simulink model "ThdRwRtStCalib"  (R2024b)
settings: Solver=FixedStepDiscrete  StartTime=0.0  StopTime=10.0  FixedStep=0.01  RelTol=1e-3
model workspace (MAT data in the model file):
  KeSMSwAcsMd7ThdRwRtStBkReclnUpwdDnwdPosMax_Val : Simulink.Parameter (value not decoded)
  KeSMSwAcsMd7ThdRwRtStBkReclnUpwdDnwdPosMin_Val : Simulink.Parameter (value not decoded)
  KeSMSwAcsMd7ThdRwRtStBkReclnUpwdDnwdPos_Val : Simulink.Parameter (value not decoded)
  KeSMSwAcsMd7ThdRwRtStCshnFldUpwdDnwdPosMax_Val : Simulink.Parameter (value not decoded)
  KeSMSwAcsMd7ThdRwRtStCshnFldUpwdDnwdPosMin_Val : Simulink.Parameter (value not decoded)
  KeSMSwAcsMd7ThdRwRtStCshnFldUpwdDnwdPos_Val : Simulink.Parameter (value not decoded)
  KeSMSwAcsMd7ThdRwRtStFrwdBkwdPosMax_Val : Simulink.Parameter (value not decoded)
  KeSMSwAcsMd7ThdRwRtStFrwdBkwdPosMin_Val : Simulink.Parameter (value not decoded)
  KeSMSwAcsMd7ThdRwRtStFrwdBkwdPos_Val : Simulink.Parameter (value not decoded)
symbols that are objects in the model workspace (value not decoded): KeSMSwAcsMd7ThdRwRtStBkReclnUpwdDnwdPos_Val, KeSMSwAcsMd7ThdRwRtStBkReclnUpwdDnwdPosMax_Val, KeSMSwAcsMd7ThdRwRtStBkReclnUpwdDnwdPosMin_Val, KeSMSwAcsMd7ThdRwRtStCshnFldUpwdDnwdPos_Val, KeSMSwAcsMd7ThdRwRtStCshnFldUpwdDnwdPosMax_Val, KeSMSwAcsMd7ThdRwRtStCshnFldUpwdDnwdPosMin_Val, KeSMSwAcsMd7ThdRwRtStFrwdBkwdPos_Val, KeSMSwAcsMd7ThdRwRtStFrwdBkwdPosMax_Val, KeSMSwAcsMd7ThdRwRtStFrwdBkwdPosMin_Val
undefined symbols (not defined in the file or in its folder): KeSMSw6sAcsEntryThdRwRtStBkReclnUpwdDnwdPos_Val, KeSMSw6sAcsEntryThdRwRtStBkReclnUpwdDnwdPosMax_Val, KeSMSw6sAcsEntryThdRwRtStBkReclnUpwdDnwdPosMin_Val, KeSMSw6sAcsEntryThdRwRtStCshnFldUpwdDnwdPos_Val, KeSMSw6sAcsEntryThdRwRtStCshnFldUpwdDnwdPosMax_Val, KeSMSw6sAcsEntryThdRwRtStCshnFldUpwdDnwdPosMin_Val, KeSMSw6sAcsEntryThdRwRtStFrwdBkwdPos_Val, KeSMSw6sAcsEntryThdRwRtStFrwdBkwdPosMax_Val, KeSMSw6sAcsEntryThdRwRtStFrwdBkwdPosMin_Val, KeSMSw6SAcsMd56ThdRwRtStBkReclnUpwdDnwdPos_Val, KeSMSw6SAcsMd56ThdRwRtStBkReclnUpwdDnwdPosMax_Val, KeSMSw6SAcsMd56ThdRwRtStBkReclnUpwdDnwdPosMin_Val, KeSMSw6SAcsMd56ThdRwRtStFrwdBkwdPos_Val, KeSMSw6SAcsMd56ThdRwRtStFrwdBkwdPosMax_Val, KeSMSw6SAcsMd56ThdRwRtStFrwdBkwdPosMin_Val, KeSMSw6SAcsMd57ThdRwRtStBkReclnUpwdDnwdPos_Val, KeSMSw6SAcsMd57ThdRwRtStBkReclnUpwdDnwdPosMax_Val, KeSMSw6SAcsMd57ThdRwRtStBkReclnUpwdDnwdPosMin_Val, KeSMSw6SAcsMd57ThdRwRtStFrwdBkwdPos_Val, KeSMSw6SAcsMd57ThdRwRtStFrwdBkwdPosMax_Val, KeSMSw6SAcsMd57ThdRwRtStFrwdBkwdPosMin_Val, KeSMSw6sFamilyMdThdRwRtStFrwdBkwdPos_Val, KeSMSw6sFamilyMdThdRwRtStFrwdBkwdPosMax_Val, KeSMSw6sFamilyMdThdRwRtStFrwdBkwdPosMin_Val, KeSMSw6sFamilyRMdThdRwRtStFrwdBkwdPos_Val, KeSMSw6sFamilyRMdThdRwRtStFrwdBkwdPosMax_Val, KeSMSw6sFamilyRMdThdRwRtStFrwdBkwdPosMin_Val, KeSMSw6sLugThdRwRtStBkReclnUpwdDnwdPos_Val, KeSMSw6sLugThdRwRtStBkReclnUpwdDnwdPosMax_Val, KeSMSw6sLugThdRwRtStBkReclnUpwdDnwdPosMin_Val, KeSMSw6sLugThdRwRtStCshnFldUpwdDnwdPos_Val, KeSMSw6sLugThdRwRtStCshnFldUpwdDnwdPosMax_Val, KeSMSw6sLugThdRwRtStCshnFldUpwdDnwdPosMin_Val, KeSMSw6sLugThdRwRtStFrwdBkwdPos_Val, KeSMSw6sLugThdRwRtStFrwdBkwdPosMax_Val, KeSMSw6sLugThdRwRtStFrwdBkwdPosMin_Val, KeSMSw6sVIPThdRwRtStBkReclnUpwdDnwdPos_Val, KeSMSw6sVIPThdRwRtStBkReclnUpwdDnwdPosMax_Val, KeSMSw6sVIPThdRwRtStBkReclnUpwdDnwdPosMin_Val, KeSMSw6sVIPThdRwRtStFrwdBkwdPos_Val, KeSMSw6sVIPThdRwRtStFrwdBkwdPosMax_Val, KeSMSw6sVIPThdRwRtStFrwdBkwdPosMin_Val, KeSMSwAcsEntryThdRwRtStBkReclnUpwdDnwdPos_Val, KeSMSwAcsEntryThdRwRtStBkReclnUpwdDnwdPosMax_Val, KeSMSwAcsEntryThdRwRtStBkReclnUpwdDnwdPosMin_Val, KeSMSwAcsEntryThdRwRtStCshnFldUpwdDnwdPos_Val, KeSMSwAcsEntryThdRwRtStCshnFldUpwdDnwdPosMax_Val, KeSMSwAcsEntryThdRwRtStCshnFldUpwdDnwdPosMin_Val, KeSMSwAcsEntryThdRwRtStFrwdBkwdPos_Val, KeSMSwAcsEntryThdRwRtStFrwdBkwdPosMax_Val, KeSMSwAcsEntryThdRwRtStFrwdBkwdPosMin_Val, KeSMSwAcsMd53ThdRwRtBkReclnUpwdDnwdPos_Val, KeSMSwAcsMd53ThdRwRtBkReclnUpwdDnwdPosMax_Val, KeSMSwAcsMd53ThdRwRtBkReclnUpwdDnwdPosMin_Val, KeSMSwAcsMd53ThdRwRtFldUpwdDnwdPos_Val, KeSMSwAcsMd53ThdRwRtFldUpwdDnwdPosMax_Val, KeSMSwAcsMd53ThdRwRtFldUpwdDnwdPosMin_Val, KeSMSwAcsMd56ThdRwRtStBkReclnUpwdDnwdPos_Val, KeSMSwAcsMd56ThdRwRtStBkReclnUpwdDnwdPosMax_Val, KeSMSwAcsMd56ThdRwRtStBkReclnUpwdDnwdPosMin_Val ... (+33)
libraries: TrgtPosSelcLib x18
(part 3 of 3)

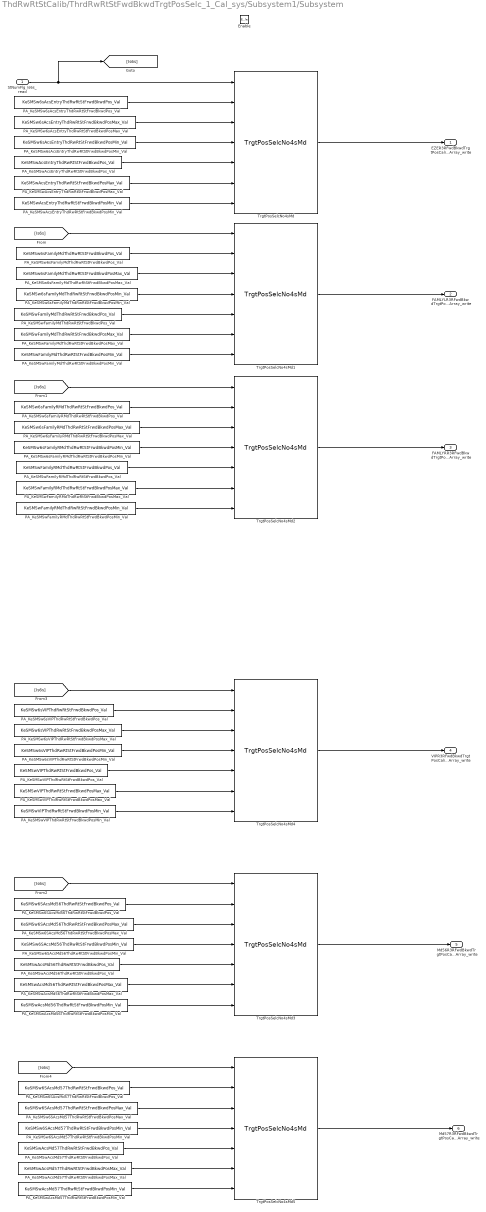
== system ThdRwRtStCalib/ThrdRwRtStFwdBkwdTrgtPosSelc_1_Cal_sys/Subsystem1/Subsystem ==
  StNumFlg_Is6s_read : Inport
  Enable : EnablePort
  PA_KeSMSw6SAcsMd56ThdRwRtStFrwdBkwdPosMax_Val : Constant  Value=KeSMSw6SAcsMd56ThdRwRtStFrwdBkwdPosMax_Val
  PA_KeSMSw6SAcsMd56ThdRwRtStFrwdBkwdPosMin_Val : Constant  Value=KeSMSw6SAcsMd56ThdRwRtStFrwdBkwdPosMin_Val
  PA_KeSMSw6SAcsMd56ThdRwRtStFrwdBkwdPos_Val : Constant  Value=KeSMSw6SAcsMd56ThdRwRtStFrwdBkwdPos_Val
  PA_KeSMSw6SAcsMd57ThdRwRtStFrwdBkwdPosMax_Val : Constant  Value=KeSMSw6SAcsMd57ThdRwRtStFrwdBkwdPosMax_Val
  PA_KeSMSw6SAcsMd57ThdRwRtStFrwdBkwdPosMin_Val : Constant  Value=KeSMSw6SAcsMd57ThdRwRtStFrwdBkwdPosMin_Val
  PA_KeSMSw6SAcsMd57ThdRwRtStFrwdBkwdPos_Val : Constant  Value=KeSMSw6SAcsMd57ThdRwRtStFrwdBkwdPos_Val
  PA_KeSMSw6sAcsEntryThdRwRtStFrwdBkwdPosMax_Val : Constant  Value=KeSMSw6sAcsEntryThdRwRtStFrwdBkwdPosMax_Val
  PA_KeSMSw6sAcsEntryThdRwRtStFrwdBkwdPosMin_Val : Constant  Value=KeSMSw6sAcsEntryThdRwRtStFrwdBkwdPosMin_Val
  PA_KeSMSw6sAcsEntryThdRwRtStFrwdBkwdPos_Val : Constant  Value=KeSMSw6sAcsEntryThdRwRtStFrwdBkwdPos_Val
  PA_KeSMSw6sFamilyMdThdRwRtStFrwdBkwdPosMax_Val : Constant  Value=KeSMSw6sFamilyMdThdRwRtStFrwdBkwdPosMax_Val
  PA_KeSMSw6sFamilyMdThdRwRtStFrwdBkwdPosMin_Val : Constant  Value=KeSMSw6sFamilyMdThdRwRtStFrwdBkwdPosMin_Val
  PA_KeSMSw6sFamilyMdThdRwRtStFrwdBkwdPos_Val : Constant  Value=KeSMSw6sFamilyMdThdRwRtStFrwdBkwdPos_Val
  PA_KeSMSw6sFamilyRMdThdRwRtStFrwdBkwdPosMax_Val : Constant  Value=KeSMSw6sFamilyRMdThdRwRtStFrwdBkwdPosMax_Val
  PA_KeSMSw6sFamilyRMdThdRwRtStFrwdBkwdPosMin_Val : Constant  Value=KeSMSw6sFamilyRMdThdRwRtStFrwdBkwdPosMin_Val
  PA_KeSMSw6sFamilyRMdThdRwRtStFrwdBkwdPos_Val : Constant  Value=KeSMSw6sFamilyRMdThdRwRtStFrwdBkwdPos_Val
  PA_KeSMSw6sVIPThdRwRtStFrwdBkwdPosMax_Val : Constant  Value=KeSMSw6sVIPThdRwRtStFrwdBkwdPosMax_Val
  PA_KeSMSw6sVIPThdRwRtStFrwdBkwdPosMin_Val : Constant  Value=KeSMSw6sVIPThdRwRtStFrwdBkwdPosMin_Val
  PA_KeSMSw6sVIPThdRwRtStFrwdBkwdPos_Val : Constant  Value=KeSMSw6sVIPThdRwRtStFrwdBkwdPos_Val
  PA_KeSMSwAcsEntryThdRwRtStFrwdBkwdPosMax_Val : Constant  Value=KeSMSwAcsEntryThdRwRtStFrwdBkwdPosMax_Val
  PA_KeSMSwAcsEntryThdRwRtStFrwdBkwdPosMin_Val : Constant  Value=KeSMSwAcsEntryThdRwRtStFrwdBkwdPosMin_Val
  PA_KeSMSwAcsEntryThdRwRtStFrwdBkwdPos_Val : Constant  Value=KeSMSwAcsEntryThdRwRtStFrwdBkwdPos_Val
  PA_KeSMSwAcsMd56ThdRwRtStFrwdBkwdPosMax_Val : Constant  Value=KeSMSwAcsMd56ThdRwRtStFrwdBkwdPosMax_Val
  PA_KeSMSwAcsMd56ThdRwRtStFrwdBkwdPosMin_Val : Constant  Value=KeSMSwAcsMd56ThdRwRtStFrwdBkwdPosMin_Val
  PA_KeSMSwAcsMd56ThdRwRtStFrwdBkwdPos_Val : Constant  Value=KeSMSwAcsMd56ThdRwRtStFrwdBkwdPos_Val
  PA_KeSMSwAcsMd57ThdRwRtStFrwdBkwdPosMax_Val : Constant  Value=KeSMSwAcsMd57ThdRwRtStFrwdBkwdPosMax_Val
  PA_KeSMSwAcsMd57ThdRwRtStFrwdBkwdPosMin_Val : Constant  Value=KeSMSwAcsMd57ThdRwRtStFrwdBkwdPosMin_Val
  PA_KeSMSwAcsMd57ThdRwRtStFrwdBkwdPos_Val : Constant  Value=KeSMSwAcsMd57ThdRwRtStFrwdBkwdPos_Val
  PA_KeSMSwFamilyMdThdRwRtStFrwdBkwdPosMax_Val : Constant  Value=KeSMSwFamilyMdThdRwRtStFrwdBkwdPosMax_Val
  PA_KeSMSwFamilyMdThdRwRtStFrwdBkwdPosMin_Val : Constant  Value=KeSMSwFamilyMdThdRwRtStFrwdBkwdPosMin_Val
  PA_KeSMSwFamilyMdThdRwRtStFrwdBkwdPos_Val : Constant  Value=KeSMSwFamilyMdThdRwRtStFrwdBkwdPos_Val
  PA_KeSMSwFamilyRMdThdRwRtStFrwdBkwdPosMax_Val : Constant  Value=KeSMSwFamilyRMdThdRwRtStFrwdBkwdPosMax_Val
  PA_KeSMSwFamilyRMdThdRwRtStFrwdBkwdPosMin_Val : Constant  Value=KeSMSwFamilyRMdThdRwRtStFrwdBkwdPosMin_Val
  PA_KeSMSwFamilyRMdThdRwRtStFrwdBkwdPos_Val : Constant  Value=KeSMSwFamilyRMdThdRwRtStFrwdBkwdPos_Val
  PA_KeSMSwVIPThdRwRtStFrwdBkwdPosMax_Val : Constant  Value=KeSMSwVIPThdRwRtStFrwdBkwdPosMax_Val
  PA_KeSMSwVIPThdRwRtStFrwdBkwdPosMin_Val : Constant  Value=KeSMSwVIPThdRwRtStFrwdBkwdPosMin_Val
  PA_KeSMSwVIPThdRwRtStFrwdBkwdPos_Val : Constant  Value=KeSMSwVIPThdRwRtStFrwdBkwdPos_Val
  TrgtPosSelcNo4sMd{,1..5} (6 alike) : TrgtPosSelcLib/TrgtPosSelcNo4sMd  SystemSampleTime=-1  VariantActivationTime=update diagram  AllowFlexibleInterface=on  Latency=0  AutoFrameSizeCalculation=off
  EZER3RFwdBkwdTrgtPosCalib_TrgtPosArray_write : Outport  VectorParamsAs1DForOutWhenUnconnected=off
      settings: EnsureOutportIsVirtual=on
  FAMLYLR3RFwdBkwdTrgtPosCalib_TrgtPosArray_write : Outport  Port=2  VectorParamsAs1DForOutWhenUnconnected=off
      settings: EnsureOutportIsVirtual=on
  FAMLYRR3RFwdBkwdTrgtPosCalib_TrgtPosArray_write : Outport  Port=3  VectorParamsAs1DForOutWhenUnconnected=off
      settings: EnsureOutportIsVirtual=on
  VIPR3RFwdBkwdTrgtPosCalib_TrgtPosArray_write : Outport  Port=4  VectorParamsAs1DForOutWhenUnconnected=off
      settings: EnsureOutportIsVirtual=on
  Md56R3RFwdBkwdTrgtPosCalib_TrgtPosArray_write : Outport  Port=5  VectorParamsAs1DForOutWhenUnconnected=off
      settings: EnsureOutportIsVirtual=on
  Md57R3RFwdBkwdTrgtPosCalib_TrgtPosArray_write : Outport  Port=6  VectorParamsAs1DForOutWhenUnconnected=off
      settings: EnsureOutportIsVirtual=on
  wires:
  StNumFlg_Is6s_read/1 -> [Is6s], TrgtPosSelcNo4sMd/1
  [Is6s] -> TrgtPosSelcNo4sMd1/1
  [Is6s] -> TrgtPosSelcNo4sMd2/1
  [Is6s] -> TrgtPosSelcNo4sMd4/1
  PA_KeSMSw6sAcsEntryThdRwRtStFrwdBkwdPosMax_Val/1 -> TrgtPosSelcNo4sMd/3
  PA_KeSMSw6sAcsEntryThdRwRtStFrwdBkwdPos_Val/1 -> TrgtPosSelcNo4sMd/2
  PA_KeSMSw6sAcsEntryThdRwRtStFrwdBkwdPosMin_Val/1 -> TrgtPosSelcNo4sMd/4
  PA_KeSMSw6sFamilyMdThdRwRtStFrwdBkwdPosMax_Val/1 -> TrgtPosSelcNo4sMd1/3
  PA_KeSMSw6sFamilyMdThdRwRtStFrwdBkwdPos_Val/1 -> TrgtPosSelcNo4sMd1/2
  PA_KeSMSw6sFamilyMdThdRwRtStFrwdBkwdPosMin_Val/1 -> TrgtPosSelcNo4sMd1/4
  PA_KeSMSw6sFamilyRMdThdRwRtStFrwdBkwdPosMax_Val/1 -> TrgtPosSelcNo4sMd2/3
  PA_KeSMSw6sFamilyRMdThdRwRtStFrwdBkwdPosMin_Val/1 -> TrgtPosSelcNo4sMd2/4
  PA_KeSMSw6sFamilyRMdThdRwRtStFrwdBkwdPos_Val/1 -> TrgtPosSelcNo4sMd2/2
  PA_KeSMSw6sVIPThdRwRtStFrwdBkwdPosMax_Val/1 -> TrgtPosSelcNo4sMd4/3
  PA_KeSMSw6sVIPThdRwRtStFrwdBkwdPos_Val/1 -> TrgtPosSelcNo4sMd4/2
  PA_KeSMSw6sVIPThdRwRtStFrwdBkwdPosMin_Val/1 -> TrgtPosSelcNo4sMd4/4
  PA_KeSMSwAcsEntryThdRwRtStFrwdBkwdPosMax_Val/1 -> TrgtPosSelcNo4sMd/6
  PA_KeSMSwAcsEntryThdRwRtStFrwdBkwdPos_Val/1 -> TrgtPosSelcNo4sMd/5
  PA_KeSMSwAcsEntryThdRwRtStFrwdBkwdPosMin_Val/1 -> TrgtPosSelcNo4sMd/7
  PA_KeSMSwFamilyMdThdRwRtStFrwdBkwdPosMax_Val/1 -> TrgtPosSelcNo4sMd1/6
  PA_KeSMSwFamilyMdThdRwRtStFrwdBkwdPos_Val/1 -> TrgtPosSelcNo4sMd1/5
  PA_KeSMSwFamilyMdThdRwRtStFrwdBkwdPosMin_Val/1 -> TrgtPosSelcNo4sMd1/7
  PA_KeSMSwFamilyRMdThdRwRtStFrwdBkwdPosMax_Val/1 -> TrgtPosSelcNo4sMd2/6
  PA_KeSMSwFamilyRMdThdRwRtStFrwdBkwdPos_Val/1 -> TrgtPosSelcNo4sMd2/5
  PA_KeSMSwFamilyRMdThdRwRtStFrwdBkwdPosMin_Val/1 -> TrgtPosSelcNo4sMd2/7
  PA_KeSMSwVIPThdRwRtStFrwdBkwdPosMax_Val/1 -> TrgtPosSelcNo4sMd4/6
  PA_KeSMSwVIPThdRwRtStFrwdBkwdPos_Val/1 -> TrgtPosSelcNo4sMd4/5
  PA_KeSMSwVIPThdRwRtStFrwdBkwdPosMin_Val/1 -> TrgtPosSelcNo4sMd4/7
  TrgtPosSelcNo4sMd/1 -> EZER3RFwdBkwdTrgtPosCalib_TrgtPosArray_write/1
  TrgtPosSelcNo4sMd1/1 -> FAMLYLR3RFwdBkwdTrgtPosCalib_TrgtPosArray_write/1
  TrgtPosSelcNo4sMd2/1 -> FAMLYRR3RFwdBkwdTrgtPosCalib_TrgtPosArray_write/1
  TrgtPosSelcNo4sMd4/1 -> VIPR3RFwdBkwdTrgtPosCalib_TrgtPosArray_write/1
  [Is6s] -> TrgtPosSelcNo4sMd3/1
  PA_KeSMSw6SAcsMd56ThdRwRtStFrwdBkwdPos_Val/1 -> TrgtPosSelcNo4sMd3/2
  PA_KeSMSw6SAcsMd56ThdRwRtStFrwdBkwdPosMax_Val/1 -> TrgtPosSelcNo4sMd3/3
  PA_KeSMSw6SAcsMd56ThdRwRtStFrwdBkwdPosMin_Val/1 -> TrgtPosSelcNo4sMd3/4
  PA_KeSMSwAcsMd56ThdRwRtStFrwdBkwdPos_Val/1 -> TrgtPosSelcNo4sMd3/5
  PA_KeSMSwAcsMd56ThdRwRtStFrwdBkwdPosMin_Val/1 -> TrgtPosSelcNo4sMd3/7
  PA_KeSMSwAcsMd56ThdRwRtStFrwdBkwdPosMax_Val/1 -> TrgtPosSelcNo4sMd3/6
  TrgtPosSelcNo4sMd3/1 -> Md56R3RFwdBkwdTrgtPosCalib_TrgtPosArray_write/1
  TrgtPosSelcNo4sMd5/1 -> Md57R3RFwdBkwdTrgtPosCalib_TrgtPosArray_write/1
  [Is6s] -> TrgtPosSelcNo4sMd5/1
  PA_KeSMSw6SAcsMd57ThdRwRtStFrwdBkwdPosMax_Val/1 -> TrgtPosSelcNo4sMd5/3
  PA_KeSMSw6SAcsMd57ThdRwRtStFrwdBkwdPos_Val/1 -> TrgtPosSelcNo4sMd5/2
  PA_KeSMSw6SAcsMd57ThdRwRtStFrwdBkwdPosMin_Val/1 -> TrgtPosSelcNo4sMd5/4
  PA_KeSMSwAcsMd57ThdRwRtStFrwdBkwdPosMax_Val/1 -> TrgtPosSelcNo4sMd5/6
  PA_KeSMSwAcsMd57ThdRwRtStFrwdBkwdPos_Val/1 -> TrgtPosSelcNo4sMd5/5
  PA_KeSMSwAcsMd57ThdRwRtStFrwdBkwdPosMin_Val/1 -> TrgtPosSelcNo4sMd5/7
